simulink model "sysgenQAM16"  (Simulink 7.3)
settings: Solver=ode45  StartTime=0.0  StopTime=5000  RelTol=1e-3
PreLoadFcn:
  | xlrequire('PreLoadFcn')
values from neighbouring files (symbols this model uses):
  hh = hh1/max(hh1)    [sysgenCostasLoop_PreLoadFcn.m]
  j = find(xLabel==')')    [sdspfscope2_r13.m]
  k = (k-1)*3+2    [sdspfscope2_r13.m]
  mu = xfix({xlSigned, 18, 15, xlRound, xlSaturate}, mu)    [lmsErr.m]
undefined symbols (not defined in the file or in its folder): chan, k_i0, k_p0, xlipgetpartsetting, xlsfunxy
libraries: xbsIndex_r4 x263, dspmlti4 x2, dspsigops x2, dspbuff3 x1, xbsCopyrightNotice_r4 x1, dspobslib x1, simulink x1, dspsnks4 x1
(part 1 of 4)
settings Model: Creator=alexc  LastModifiedBy=douangp  ExtModeTrigMode=oneshot  ExtModeArmWhenConnect=off
settings DataIOCC: LimitDataPoints=off  SignalLoggingName=sigsOut
settings OptimizationCC: BlockReduction=off  BooleanDataType=off  InlineInvariantSignals=on  InitFltsAndDblsToZero=on
settings DebuggingCC: SaveWithParameterizedLinksMsg=none  SignalResolutionControl=TryResolveAllWithWarning  SolverPrmCheckMsg=none  MultiTaskDSMMsg=warning  MultiTaskCondExecSysMsg=none  StrictBusMsg=None
settings HardwareCC: TargetUnknown=on
settings RTWCC: IncludeERTFirstTime=on
settings GRTTargetCC: TargetFcnLib=ansi_tfl_tmw.mat

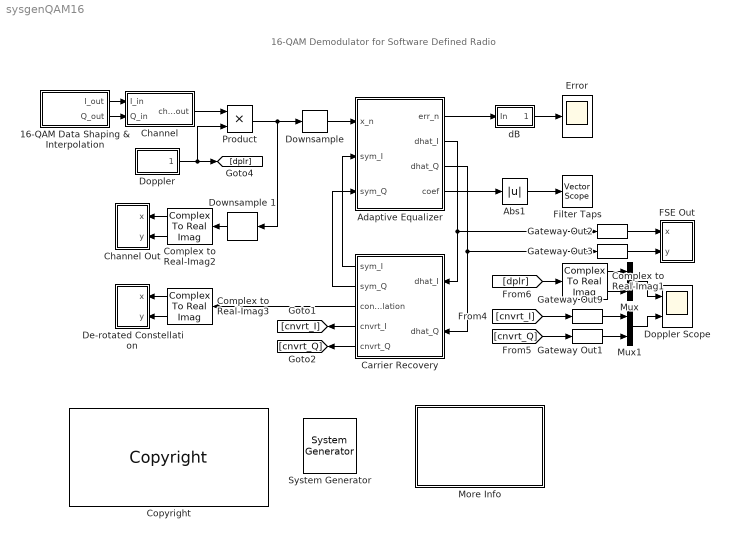
== system sysgenQAM16 ==
  note: 16-QAM Demodulator for Software Defined Radio
  " System Generator" : xbsIndex_r4/ System Generator  Tag=genX  SystemSampleTime=-1  xilinxfamily=virtex6  part=xc6vlx240t  speed=-1  package=ff784  synthesis_tool=XST  clock_wrapper=Clock Enables  directory=./netlist  testbench=off  simulink_period=1  sysclk_period=50  dcm_input_clock_period=100  incr_netlist=off  trim_vbits=Everywhere in SubSystem  dbl_ovrd=According to Block Masks  core_generation=According to Block Masks  run_coregen=off  deprecated_control=off  eval_field=0  block_type=sysgen
      settings: block_version=9.1-beta
  16-QAM Data Shaping & Interpolation : Subsystem
  Abs1 : Abs  SaturateOnIntegerOverflow=on
  Adaptive Equalizer : Subsystem
  Carrier Recovery : Subsystem
  Channel : Subsystem
  Channel Out : Subsystem  LoadFcn=xlsfunxy([],[],[],'LoadBlock')  StartFcn=xlsfunxy([],[],[],'Start')  StopFcn=xlsfunxy([],[],[],'Stop')  mask(My XY scope.){xmin=-2.25, xmax=2.25, ymin=-2.25, ymax=2.25, refresh=800, style='.', st=-1}
      mask prompts: xmin "x-min:"; xmax "x-max:"; ymin "y-min:"; ymax "y-max:"; refresh "Refresh rate"; style "Line/Marker style"; st "Sample time:"
      mask help: XY scope using MATLAB graph window. First input is used as time base. Enter plotting ranges.
      settings: CopyFcn=xlsfunxy([],[],[],'CopyBlock')  DeleteFcn=xlsfunxy([],[],[],'DeleteBlock')  NameChangeFcn=xlsfunxy([],[],[],'NameChange')
      mask Help: This block can be used to explore limit cycles. Look at the m-file xlsfunxy.m to see how it works.
      mask Display: plot([.05 .95 .95 .05 .05],[.45 .45 .95 .95 .45], 0.5+cos(0:0.1:2*pi)*0.3,0.7+sin(0:0.1:2*pi)*0.2)
  Complex to Real-Imag1 : ComplexToRealImag
  Complex to Real-Imag2 : ComplexToRealImag
  Complex to Real-Imag3 : ComplexToRealImag
  Copyright : xbsCopyrightNotice_r4/Copyright  copyrighttext="Copyright (c) 2009  by  Xilinx, Inc. All rights reserved.<br><br>This file contains proprietary, confidential information of Xilinx, Inc., is distributed under licensefrom Xilinx, Inc., and may be used, copied and/or disclosed only pursuant to the terms of a valid licenseagreement with Xilinx, Inc. Xilinx hereby grants you a license to use this file solely for design,simulation, implementation and creation of design files limited to Xilinx devices or technologies. Use with non-Xilinx devices or technologies is expressly prohibited and immediately terminates your license unless covered by a separate agreement.<br><br>Xilinx is providing this design, code, or information \"as-is\" solely for use in developing programs and solutions for Xilinx devices, with no obligation on the part of Xilinx to provide support. By providingthis design, code, or information as one possible implementation of this feature, application or standard,Xilinx is making no representation that this implementation is free from any claims of infringement. Youare responsible for obtaining any rights you may require for your implementation. Xilinx expressly disclaimsany warranty whatsoever with respect to the adequacy of the implementation, including but not limited to anywarranties or representations that this implementation is free from claims of infringement, implied warrantiesof merchantability or fitness for a particular purpose.<br><br>Xilinx products are not intended for use in life support appliances, devices, or systems. Use in such applications is expressly prohibited.<br><br>Any modifications that are made to the Source Code are done at the user's sole risk and will be unsupported.<br><br>This copyright and support notice must be retained as part of this text at all times. (c) Copyright 1995-2009 Xilinx, Inc. All rights reserved."  block_type=copyright
      settings: block_version=10.1.00
      settings: infoedit=|
      | Copyright(C) 2008 by  Xilinx, Inc. All rights reserved.<br>
      | <br>
      | This file contains proprietary, confidential information of Xilinx, Inc., is distributed under license
      | from Xilinx, Inc., and may be used, copied and/or disclosed only pursuant to the terms of a valid license
      | agreement with Xilinx, Inc. Xilinx hereby grants you a license to use this file solely for design,
      | simulation, implementation and creation of design files limited to Xilinx devices or technologies. Use
      | with non-Xilinx devices or technologies is expressly prohibited and immediately terminates your license
      | unless covered by a separate agreement.<br>
      | <br>
      | Xilinx is providing this design, code, or information "as-is" solely for use in developing programs and
      | solutions for Xilinx devices, with no obligation on the part of Xilinx to provide support. By providing
      | this design, code, or information as one possible implementation of this feature, application or standard,
      | Xilinx is making no representation that this implementation is free from any claims of infringement. You
      | are responsible for obtaining any rights you may require for your implementation. Xilinx expressly disclaims
      | any warranty whatsoever with respect to the adequacy of the implementation, including but not limited to any
      | warranties or representations that this implementation is free from claims of infringement, implied warranties
      | of merchantability or fitness for a particular purpose.<br>
      | <br>
      | Xilinx products are not intended for use in life support appliances, devices, or systems. Use in such
      | applications is expressly prohibited.<br>
      | <br>
      | Any modifications that are made to the Source Code are done at the user's sole risk and will be unsupported.<br>
      | <br>
      | This copyright and support notice must be retained as part of this text at all times.
      | (c) Copyright 1995-2008 Xilinx, Inc. All rights reserved.
  De-rotated Constellation : Subsystem  LoadFcn=xlsfunxy([],[],[],'LoadBlock')  StartFcn=xlsfunxy([],[],[],'Start')  StopFcn=xlsfunxy([],[],[],'Stop')  mask(My XY scope.){xmin=-1.5, xmax=1.5, ymin=-1.5, ymax=1.5, refresh=800, style='.', st=-1}
      mask prompts: xmin "x-min:"; xmax "x-max:"; ymin "y-min:"; ymax "y-max:"; refresh "Refresh rate"; style "Line/Marker style"; st "Sample time:"
      mask help: XY scope using MATLAB graph window. First input is used as time base. Enter plotting ranges.
      settings: CopyFcn=xlsfunxy([],[],[],'CopyBlock')  DeleteFcn=xlsfunxy([],[],[],'DeleteBlock')  NameChangeFcn=xlsfunxy([],[],[],'NameChange')
      mask Help: This block can be used to explore limit cycles. Look at the m-file xlsfunxy.m to see how it works.
      mask Display: plot([.05 .95 .95 .05 .05],[.45 .45 .95 .95 .45], 0.5+cos(0:0.1:2*pi)*0.3,0.7+sin(0:0.1:2*pi)*0.2)
  Doppler : Subsystem
  Doppler Scope : Scope  NumInputPorts=2
      settings: TimeRange=4000  YMin=-1~-1  YMax=1~1
  "Downsample " : dspsigops/Downsample  N=2  phase=0  ic=0  smode=Allow multirate  fmode=Maintain input frame size
  Downsample 1 : dspsigops/Downsample  N=4  phase=0  ic=0  smode=Allow multirate  fmode=Maintain input frame size
  Error : Scope
      settings: TimeRange=500  YMin=-60  YMax=-22.5
  FSE Out : Subsystem  LoadFcn=xlsfunxy([],[],[],'LoadBlock')  StartFcn=xlsfunxy([],[],[],'Start')  StopFcn=xlsfunxy([],[],[],'Stop')  mask(My XY scope.){xmin=-2.25, xmax=2.25, ymin=-2.25, ymax=2.25, refresh=800, style='.', st=-1}
      mask prompts: xmin "x-min:"; xmax "x-max:"; ymin "y-min:"; ymax "y-max:"; refresh "Refresh rate"; style "Line/Marker style"; st "Sample time:"
      mask help: XY scope using MATLAB graph window. First input is used as time base. Enter plotting ranges.
      settings: CopyFcn=xlsfunxy([],[],[],'CopyBlock')  DeleteFcn=xlsfunxy([],[],[],'DeleteBlock')  NameChangeFcn=xlsfunxy([],[],[],'NameChange')
      mask Help: This block can be used to explore limit cycles. Look at the m-file xlsfunxy.m to see how it works.
      mask Display: plot([.05 .95 .95 .05 .05],[.45 .45 .95 .95 .45], 0.5+cos(0:0.1:2*pi)*0.3,0.7+sin(0:0.1:2*pi)*0.2)
  Filter Taps : dspsnks4/Vector Scope  DialogController=dspdialog.VectorScope  DialogControllerArgs=DataTag3  ScopeProperties=on  Domain=User-defined  HorizSpan=1  DisplayProperties=off  AxisGrid=on  Memory=off  FrameNumber=on  AxisLegend=off  AxisZoom=on  OpenScopeAtSimStart=on  OpenScopeImmediately=off  FigPos=[66 260 329 270]  AxisProperties=off  XUnits=Hertz  XRange=[0...Fs/2]  InheritXIncr=on  XIncr=1  XLabel=Samples  XLimit=Auto  XMin=0  XMax=1  XStart=0  YUnits=dB  YLabel=Filter Coefficients  LineProperties=off  LineDisables=on  LineStyles=:  LineMarkers=.  LineColors=[0 0 1]  XAxisParamsVer=6.8
      settings: YMin=0.00597900340780036  YMax=1.03689353636578
  Gateway Out{1..3,9} (4 alike) : xbsIndex_r4/Gateway Out  hdl_port=off  timing_constraint=None  locs_specified=off  LOCs={}  block_type=gatewayout
      settings: infoedit="Gateway out block.  Converts Xilinx fixed point inputs into ouputs of type Simulink integer, double, or fixed point.<P><P>Hardware notes:  In hardware these blocks become top level output ports or are discarded, depending on how they are configured."  xl_area=[0 0 0 0 0 0 0]  block_version=VER_STRING_GOES_HERE
  More Info : Subsystem
      mask Display: disp('Double click\n for\n more information.')
  Mux : Mux  Inputs=2
  Mux1 : Mux  Inputs=2
  Product : Product  OutDataType=sfix(16)  OutScaling=2^0  SaturateOnIntegerOverflow=on  InputSameDT=on  OutDataTypeStr=Inherit: Same as first input
  dB : Subsystem
  wires:
  16-QAM Data Shaping & Interpolation/1(I_out) -> Channel/1(I_in)
  "Downsample "/1 -> Adaptive Equalizer/1(x_n)
  16-QAM Data Shaping & Interpolation/2(Q_out) -> Channel/2(Q_in)
  Channel/1(chan_out) -> Product/1
  dB/1(Out) -> Error/1
  Gateway Out9/1 -> Mux1/1
  Gateway Out1/1 -> Mux1/2
  Mux1/1 -> Doppler Scope/2
  Complex to Real-Imag1/2 -> Mux/2
  Complex to Real-Imag1/1 -> Mux/1
  Mux/1 -> Doppler Scope/1
  [cnvrt_Q] -> Gateway Out1/1
  [dplr] -> Complex to Real-Imag1/1
  Doppler/1(doppler) -> [dplr], Product/2
  [cnvrt_I] -> Gateway Out9/1
  Adaptive Equalizer/2(dhat_I) -> Carrier Recovery/1(dhat_I), Gateway Out2/1
  Adaptive Equalizer/3(dhat_Q) -> Carrier Recovery/2(dhat_Q), Gateway Out3/1
  Carrier Recovery/1(sym_I) -> Adaptive Equalizer/2(sym_I)
  Carrier Recovery/2(sym_Q) -> Adaptive Equalizer/3(sym_Q)
  Carrier Recovery/4(cnvrt_I) -> [cnvrt_I]
  Carrier Recovery/5(cnvrt_Q) -> [cnvrt_Q]
  Complex to Real-Imag3/1 -> De-rotated Constellation/1(x)
  Complex to Real-Imag3/2 -> De-rotated Constellation/2(y)
  Carrier Recovery/3(constellation) -> Complex to Real-Imag3/1
  Product/1 -> "Downsample "/1, Downsample 1/1
  Adaptive Equalizer/1(err_n) -> dB/1(In)
  Adaptive Equalizer/4(coef) -> Abs1/1
  Abs1/1 -> Filter Taps/1
  Downsample 1/1 -> Complex to Real-Imag2/1
  Complex to Real-Imag2/2 -> Channel Out/2(y)
  Complex to Real-Imag2/1 -> Channel Out/1(x)
  Gateway Out2/1 -> FSE Out/1(x)
  Gateway Out3/1 -> FSE Out/2(y)

== system sysgenQAM16/16-QAM Data Shaping & Interpolation ==
  Complex to Real-Imag5 : ComplexToRealImag
  "FIR  Interpolation " : dspmlti4/FIR Interpolation  DialogController=dspdialog.FIRInterpolation  DialogControllerArgs=DataTag1  h=[hh]  L=4  framing=Maintain input frame size  outputBufInitCond=0  roundingMode=Floor  overflowMode=off  FilterSource=Specify via dialog  FilterObject=Hm_firinterp
  FIR  Interpolation 1 : dspmlti4/FIR Interpolation  DialogController=dspdialog.FIRInterpolation  DialogControllerArgs=DataTag2  h=[hh]  L=4  framing=Maintain input frame size  outputBufInitCond=0  roundingMode=Floor  overflowMode=off  FilterSource=Specify via dialog  FilterObject=Hm_firinterp
  QAM16 Source : Subsystem
  I_out : Outport  OutDataType=sfix(16)  OutScaling=2^0
  Q_out : Outport  Port=2  OutDataType=sfix(16)  OutScaling=2^0
  wires:
  Complex to Real-Imag5/1 -> "FIR  Interpolation "/1
  Complex to Real-Imag5/2 -> FIR  Interpolation 1/1
  QAM16 Source/1(random_data) -> Complex to Real-Imag5/1
  "FIR  Interpolation "/1 -> I_out/1
  FIR  Interpolation 1/1 -> Q_out/1

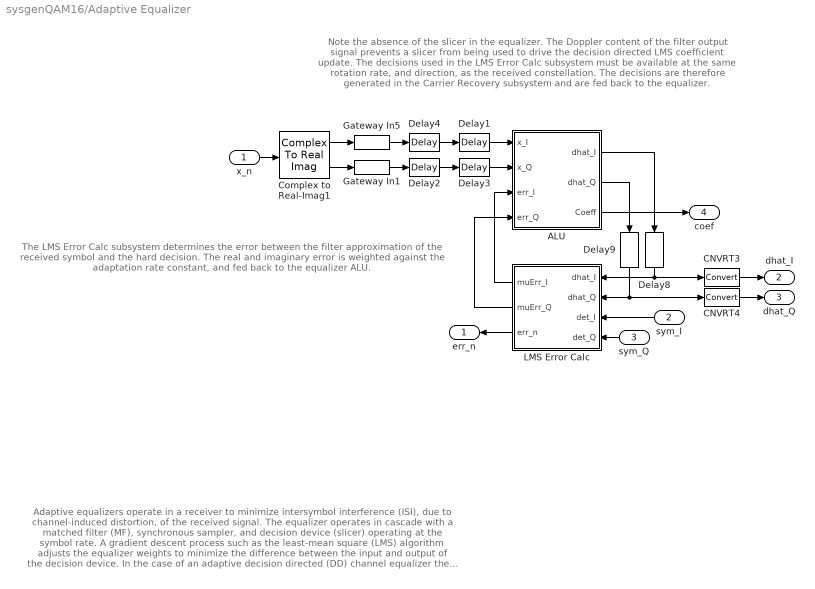
== system sysgenQAM16/Adaptive Equalizer ==
  note: Adaptive equalizers operate in a receiver to minimize intersymbol interference (ISI), due to
      | channel-induced distortion, of the received signal. The equalizer operates in cascade with
      | a matched filter (MF), synchronous sampler, and decision device (slicer) operating at the
      | symbol rate. A gradient descent process such as the least-mean square (LMS) algorithm
      | adjusts the equalizer weights to minimize the difference between the input and output of
      | the decision device.
      |
      | In the case of an adaptive decision directed (DD) channel equalizer the desired signal is
      | produced by utilizing the known structure of the system alphabet.  A 8-tap decision directed
      | equalizer using an LMS coefficient update is used in this model. The input samples are
      | complex valued quantities as are the filter weights and the output signal.
      |
      | A fractionally spaced equalizer (FSE) sampling at a rate of two samples per symbol is
      | used to avoid aliasing.  The equalizer is a multirate structure that is most efficiently
      | implemented using a polyphase decimator architecture.  For this model, two
      | polyphase arms are used.
      |
      | Additional information on adaptive equalizers and FSE can be found at:
      |
      | Haykin, S. "Adaptive Filter Theory"  Prentice Hall, New Jersey, 1996.
      |
      | J.R. Treichler, I. Fijalkow, and C.R. Johnson, Jr.  "Fractionally Spaced
      | Equalizers"  IEEE Signal Processing Magazine, May 1996, pp. 65-81.
  note: The LMS Error Calc subsystem determines
      | the error between the filter approximation of
      | the received symbol and the hard decision.
      | The real and imaginary error is weighted
      | against the adaptation rate constant, and fed
      | back to the equalizer ALU.
  note: Note the absence of the slicer in the equalizer.  The Doppler content
      | of the filter output signal prevents a slicer from being used to drive the
      | decision directed LMS coefficient update.  The decisions used in the
      | LMS Error Calc subsystem must be available at the same rotation rate,
      | and direction, as the received constellation.   The decisions are
      | therefore generated in the Carrier Recovery subsystem and are fed
      | back to the equalizer.
  x_n : Inport  OutDataType=sfix(16)  OutScaling=2^0
  sym_I : Inport  Port=2  OutDataType=sfix(16)  OutScaling=2^0
  sym_Q : Inport  Port=3  OutDataType=sfix(16)  OutScaling=2^0
  ALU : Subsystem
  CNVRT3 : xbsIndex_r4/Convert  arith_type="Signed  (2's comp)"  n_bits=18  bin_pt=14  quantization="Round  (unbiased: +/- Inf)"  overflow=Wrap  latency=0  dbl_ovrd=off  pipeline=off  block_type=convert
      settings: infoedit=The input is presented at the output after quantization and overflow effects.<P><P>Hardware notes: Additional hardware is used when rounding or saturation is selected and output width is less than the input width.  xl_area=[10 0 0 20 0 0 0]  block_version=VER_STRING_GOES_HERE
  CNVRT4 : xbsIndex_r4/Convert  arith_type="Signed  (2's comp)"  n_bits=18  bin_pt=14  quantization="Round  (unbiased: +/- Inf)"  overflow=Wrap  latency=0  dbl_ovrd=off  pipeline=off  block_type=convert
      settings: infoedit=The input is presented at the output after quantization and overflow effects.<P><P>Hardware notes: Additional hardware is used when rounding or saturation is selected and output width is less than the input width.  xl_area=[10 0 0 20 0 0 0]  block_version=VER_STRING_GOES_HERE
  Complex to Real-Imag1 : ComplexToRealImag
  Delay{1..4} (4 alike) : xbsIndex_r4/Delay  en=off  latency=1  dbl_ovrd=off  reg_retiming=off  block_type=delay
      settings: infoedit="Delay line having  configurable length.<P><P>Hardware notes: A delay line is a chain, each link of which is an SRL16 followed by a flip-flop. If register retiming is enabled, the delay line is a chain of flip-flops."  xl_area=[8 16 0 0 0 0 0]  block_version=VER_STRING_GOES_HERE
  Delay8 : xbsIndex_r4/Delay  en=off  latency=k-7  dbl_ovrd=off  reg_retiming=off  block_type=delay
      settings: infoedit="Delay line having  configurable length.<P><P>Hardware notes: A delay line is a chain, each link of which is an SRL16 followed by a flip-flop. If register retiming is enabled, the delay line is a chain of flip-flops."  xl_area=[12 24 0 24 0 0 0]  block_version=VER_STRING_GOES_HERE
  Delay9 : xbsIndex_r4/Delay  en=off  latency=k-7  dbl_ovrd=off  reg_retiming=off  block_type=delay
      settings: infoedit="Delay line having  configurable length.<P><P>Hardware notes: A delay line is a chain, each link of which is an SRL16 followed by a flip-flop. If register retiming is enabled, the delay line is a chain of flip-flops."  xl_area=[12 24 0 24 0 0 0]  block_version=VER_STRING_GOES_HERE
  Gateway In1 : xbsIndex_r4/Gateway In  arith_type="Signed  (2's comp)"  n_bits=xn_ni  bin_pt=xn_nf  quantization="Round  (unbiased: +/- Inf)"  overflow=Saturate  period=2  dbl_ovrd=off  timing_constraint=None  locs_specified=off  LOCs={}  block_type=gatewayin
      settings: infoedit="Gateway in block.  Converts inputs of type Simulink integer, double and fixed point to  Xilinx fixed point type.<P><P>Hardware notes:  In hardware these blocks become top level input ports."  xl_area=[0 0 0 0 16 0 0]  block_version=VER_STRING_GOES_HERE
  Gateway In5 : xbsIndex_r4/Gateway In  arith_type="Signed  (2's comp)"  n_bits=xn_ni  bin_pt=xn_nf  quantization="Round  (unbiased: +/- Inf)"  overflow=Saturate  period=2  dbl_ovrd=off  timing_constraint=None  locs_specified=off  LOCs={}  block_type=gatewayin
      settings: infoedit="Gateway in block.  Converts inputs of type Simulink integer, double and fixed point to  Xilinx fixed point type.<P><P>Hardware notes:  In hardware these blocks become top level input ports."  xl_area=[0 0 0 0 16 0 0]  block_version=VER_STRING_GOES_HERE
  LMS Error Calc : Subsystem
  err_n : Outport  OutDataType=sfix(16)  OutScaling=2^0
  dhat_I : Outport  Port=2  OutDataType=sfix(16)  OutScaling=2^0
  dhat_Q : Outport  Port=3  OutDataType=sfix(16)  OutScaling=2^0
  coef : Outport  Port=4  OutDataType=sfix(16)  OutScaling=2^0
  wires:
  ALU/2(dhat_Q) -> Delay9/1
  Complex to Real-Imag1/1 -> Gateway In5/1
  Complex to Real-Imag1/2 -> Gateway In1/1
  Gateway In5/1 -> Delay4/1
  Gateway In1/1 -> Delay2/1
  x_n/1 -> Complex to Real-Imag1/1
  Delay4/1 -> Delay1/1
  Delay2/1 -> Delay3/1
  Delay1/1 -> ALU/1(x_I)
  Delay3/1 -> ALU/2(x_Q)
  LMS Error Calc/3(err_n) -> err_n/1
  Delay9/1 -> LMS Error Calc/2(dhat_Q), CNVRT4/1
  sym_I/1 -> LMS Error Calc/3(det_I)
  sym_Q/1 -> LMS Error Calc/4(det_Q)
  LMS Error Calc/1(muErr_I) -> ALU/3(err_I)
  LMS Error Calc/2(muErr_Q) -> ALU/4(err_Q)
  ALU/1(dhat_I) -> Delay8/1
  Delay8/1 -> LMS Error Calc/1(dhat_I), CNVRT3/1
  CNVRT3/1 -> dhat_I/1
  CNVRT4/1 -> dhat_Q/1
  ALU/3(Coeff) -> coef/1

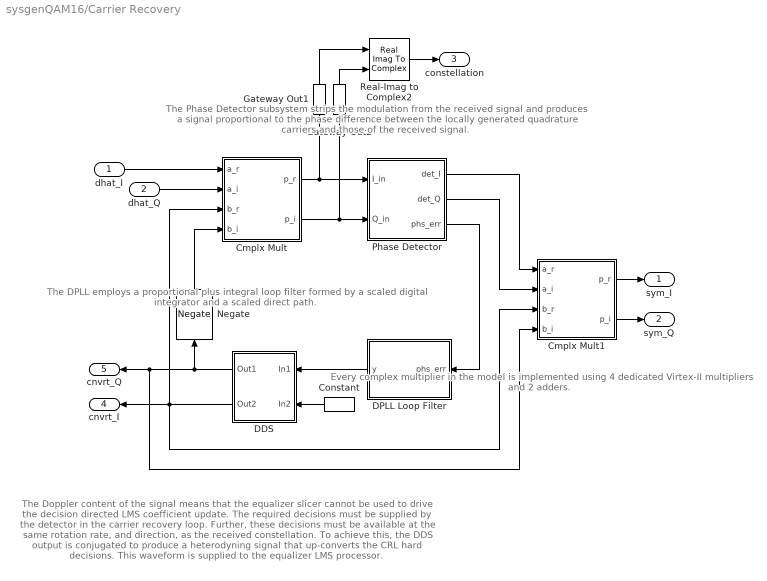
== system sysgenQAM16/Carrier Recovery ==
  note: Every complex multiplier in the model is
      | implemented using 4 dedicated Virtex-II
      | multipliers and 2 adders.
  note: The Doppler content of the signal means that the equalizer slicer cannot be used
      | to drive the decision directed LMS coefficient update.  The required decisions must
      | be supplied by the detector in the carrier recovery loop.  Further, these decisions
      | must be available at the same rotation rate, and direction, as the received constellation.
      | To achieve this, the DDS output is conjugated to produce a heterodyning signal
      | that up-converts the CRL hard decisions. This waveform is supplied to the equalizer
      | LMS processor.
  note: The Phase Detector subsystem strips the modulation
      | from the received signal and produces a signal proportional
      | to the phase difference between the locally generated
      | quadrature carriers and those of the received signal.
  note: The DPLL employs a proportional plus integral
      | loop filter formed by a scaled digital integrator
      | and a scaled direct path.
  dhat_I : Inport  OutDataType=sfix(16)  OutScaling=2^0
  dhat_Q : Inport  Port=2  OutDataType=sfix(16)  OutScaling=2^0
  Cmplx Mult : Subsystem
  Cmplx Mult1 : Subsystem
  Constant : xbsIndex_r4/Constant  arith_type=Boolean  const=1  n_bits=1  bin_pt=0  explicit_period=off  period=1  equ=P=C  opselect=C  inp2=PCIN>>17  opr=+  inp1=P  carry=CIN  dbl_ovrd=off  block_type=constant
      settings: block_version=VER_STRING_GOES_HERE
  DDS : Subsystem
  DPLL Loop Filter : Subsystem
  Gateway Out1 : xbsIndex_r4/Gateway Out  hdl_port=on  timing_constraint="Data Rate;  Set 'FAST' Attribute"  locs_specified=off  LOCs={}  block_type=gatewayout
      settings: infoedit="Gateway out block.  Converts Xilinx fixed point inputs into ouputs of type Simulink integer, double, or fixed point.<P><P>Hardware notes:  In hardware these blocks become top level output ports or are discarded, depending on how they are configured."  xl_area=[0 0 0 0 36 0 0]  block_version=VER_STRING_GOES_HERE
  Gateway Out2 : xbsIndex_r4/Gateway Out  hdl_port=on  timing_constraint="Data Rate;  Set 'FAST' Attribute"  locs_specified=off  LOCs={}  block_type=gatewayout
      settings: infoedit="Gateway out block.  Converts Xilinx fixed point inputs into ouputs of type Simulink integer, double, or fixed point.<P><P>Hardware notes:  In hardware these blocks become top level output ports or are discarded, depending on how they are configured."  xl_area=[0 0 0 0 36 0 0]  block_version=VER_STRING_GOES_HERE
  Negate : xbsIndex_r4/Negate  precision=Full  arith_type=Unsigned  n_bits=8  bin_pt=2  quantization=Truncate  overflow=Wrap  en=off  latency=0  dbl_ovrd=off  block_type=negate
      settings: xl_area=[9 0 0 17 0 0 0]  block_version=VER_STRING_GOES_HERE
  Phase Detector : Subsystem
  Real-Imag to Complex2 : RealImagToComplex
  sym_I : Outport  OutDataType=sfix(16)  OutScaling=2^0
  sym_Q : Outport  Port=2  OutDataType=sfix(16)  OutScaling=2^0
  constellation : Outport  Port=3  OutDataType=sfix(16)  OutScaling=2^0
  cnvrt_I : Outport  Port=4  OutDataType=sfix(16)  OutScaling=2^0
  cnvrt_Q : Outport  Port=5  OutDataType=sfix(16)  OutScaling=2^0
  wires:
  Cmplx Mult/1(p_r) -> Gateway Out1/1, Phase Detector/1(I_in)
  dhat_Q/1 -> Cmplx Mult/2(a_i)
  dhat_I/1 -> Cmplx Mult/1(a_r)
  Cmplx Mult/2(p_i) -> Gateway Out2/1, Phase Detector/2(Q_in)
  Gateway Out1/1 -> Real-Imag to Complex2/1
  Gateway Out2/1 -> Real-Imag to Complex2/2
  Real-Imag to Complex2/1 -> constellation/1
  Cmplx Mult1/2(p_i) -> sym_Q/1
  Phase Detector/3(phs_err) -> DPLL Loop Filter/1(phs_err)
  Phase Detector/1(det_I) -> Cmplx Mult1/1(a_r)
  Phase Detector/2(det_Q) -> Cmplx Mult1/2(a_i)
  Cmplx Mult1/1(p_r) -> sym_I/1
  DDS/2(Out2) -> Cmplx Mult/3(b_r), cnvrt_I/1, Cmplx Mult1/3(b_r)
  DDS/1(Out1) -> cnvrt_Q/1, Cmplx Mult1/4(b_i), Negate/1
  DPLL Loop Filter/1(y) -> DDS/1(In1)
  Constant/1 -> DDS/2(In2)
  Negate/1 -> Cmplx Mult/4(b_i)

== system sysgenQAM16/Channel ==
  I_in : Inport  OutDataType=sfix(16)  OutScaling=2^0
  Q_in : Inport  Port=2  OutDataType=sfix(16)  OutScaling=2^0
  Channel : Subsystem
  Channel1 : Subsystem
  Gain : Gain  Gain=j  ParameterDataType=sfix(16)  ParameterScaling=2^0  OutDataType=sfix(16)  OutScaling=2^0  SaturateOnIntegerOverflow=on  OutDataTypeStr=Inherit: Same as input  ParamDataTypeStr=Inherit: Same as input
  Sum : Sum  OutDataType=sfix(16)  OutScaling=2^0  SaturateOnIntegerOverflow=on  InputSameDT=on  OutDataTypeStr=Inherit: Same as first input
  chan_out : Outport  OutDataType=sfix(16)  OutScaling=2^0
  wires:
  Gain/1 -> Sum/2
  Channel/1(y_n) -> Sum/1
  Channel1/1(y_n) -> Gain/1
  I_in/1 -> Channel/1(x_n)
  Q_in/1 -> Channel1/1(x_n)
  Sum/1 -> chan_out/1

== system sysgenQAM16/Channel Out ==
  x : Inport  OutDataType=sfix(16)  OutScaling=2^0
  y : Inport  Port=2  OutDataType=sfix(16)  OutScaling=2^0
  Mux : Mux  Inputs=2
  xlsfunxy : S-Function  FunctionName=xlsfunxy  Parameters=[xmin xmax ymin ymax],refresh,style,st  EnableBusSupport=off
  wires:
  Mux/1 -> xlsfunxy/1
  x/1 -> Mux/1
  y/1 -> Mux/2

== system sysgenQAM16/De-rotated Constellation ==
  x : Inport  OutDataType=sfix(16)  OutScaling=2^0
  y : Inport  Port=2  OutDataType=sfix(16)  OutScaling=2^0
  Mux : Mux  Inputs=2
  xlsfunxy : S-Function  FunctionName=xlsfunxy  Parameters=[xmin xmax ymin ymax],refresh,style,st  EnableBusSupport=off
  wires:
  Mux/1 -> xlsfunxy/1
  x/1 -> Mux/1
  y/1 -> Mux/2

== system sysgenQAM16/Doppler ==
  DSP Constant : dspobslib/DSP Constant  SystemSampleTime=-1  Value=1  SampleMode=Discrete  discreteOutput=Sample-based  continuousOutput=Sample-based  sampTime=1  framePeriod=1  dataType=Inherit from 'Constant value'  isSigned=on  wordLen=16  udDataType=sfix(16)  fracBitsMode=Best precision  numFracBits=15  InterpretAs1D=off  Ts=1  FramebasedOutput=off
  Frequency Delta : simulink/Math Operations/Slider Gain  SystemSampleTime=-1  low=-0.1  gain=0.001  high=0.1
  R:I : RealImagToComplex
  TX Doppler : Subsystem
  Terminator : Terminator
  doppler : Outport  OutDataType=sfix(16)  OutScaling=2^0
  wires:
  TX Doppler/1(Cos) -> R:I/1
  TX Doppler/2(Sin) -> R:I/2
  Frequency Delta/1 -> TX Doppler/1(In1)
  DSP Constant/1 -> Frequency Delta/1
  R:I/1 -> doppler/1
  TX Doppler/3(DDS Theta) -> Terminator/1

== system sysgenQAM16/FSE Out ==
  x : Inport  OutDataType=sfix(16)  OutScaling=2^0
  y : Inport  Port=2  OutDataType=sfix(16)  OutScaling=2^0
  Mux : Mux  Inputs=2
  xlsfunxy : S-Function  FunctionName=xlsfunxy  Parameters=[xmin xmax ymin ymax],refresh,style,st  EnableBusSupport=off
  wires:
  y/1 -> Mux/2
  x/1 -> Mux/1
  Mux/1 -> xlsfunxy/1

== system sysgenQAM16/More Info ==
  note: 16-QAM Demodulator for Software Defined Radio
  note: This design implements an equalized 16-QAM demodulator for use in a software defined
      | radio.  The receiver architecture provides subsystems that demonstrate adaptive channel
      | equalization and carrier tracking on a random QAM data source.
      |
      | In addition to the System Generator demodulator components, the model includes Simulink
      | subsystems that introduce channel effects and Doppler content into the data source.  Scopes
      | are provided at important nodes for analysis purposes.  The operation of receiver is best
      | illustrated with a long simulation duration, so that the points in the de-rotated constellation
      | have sufficient time to converge.
      |
      | Additional information on software radios can be found at:
      |
      | Chris H. Dick, "Design and implementation of high-performance FPGA signal processing
      | datapaths for software-defined radios" VMEbus Systems, August 2001

== system sysgenQAM16/dB ==
  In : Inport  OutDataType=sfix(16)  OutScaling=2^0
  Abs : Abs  SaturateOnIntegerOverflow=on
  Constant : Constant  Value=0  OutDataType=sfix(16)  OutScaling=2^0
  Constant1 : Constant  OutDataType=sfix(16)  OutScaling=2^0
  Constant2 : Constant  OutDataType=sfix(16)  OutScaling=2^0
  Gain1 : Gain  Gain=20  ParameterDataType=sfix(16)  ParameterScaling=2^0  OutDataType=sfix(16)  OutScaling=2^0  SaturateOnIntegerOverflow=on  OutDataTypeStr=Inherit: Same as input  ParamDataTypeStr=Inherit: Same as input
  Multiport Switch : MultiPortSwitch  Inputs=2  SaturateOnIntegerOverflow=on  InputSameDT=on
  Relational Operator : RelationalOperator  Operator===  InputSameDT=on
  Sum : Sum  Inputs=|++  OutDataType=sfix(16)  OutScaling=2^0  SaturateOnIntegerOverflow=on  InputSameDT=on  OutDataTypeStr=Inherit: Same as first input
  log10 : Math  Operator=log10  OutDataType=sfix(16)  OutScaling=2^0  SaturateOnIntegerOverflow=on
  Out : Outport  OutDataType=sfix(16)  OutScaling=2^0
  wires:
  Multiport Switch/1 -> log10/1
  Constant1/1 -> Multiport Switch/3
  Constant/1 -> Relational Operator/1
  Abs/1 -> Multiport Switch/2, Relational Operator/2
  Constant2/1 -> Sum/2
  Sum/1 -> Multiport Switch/1
  Relational Operator/1 -> Sum/1
  Gain1/1 -> Out/1
  In/1 -> Abs/1
  log10/1 -> Gain1/1

== system sysgenQAM16/16-QAM Data Shaping & Interpolation/QAM16 Source ==
  QAM16 - I : Subsystem
  QAM16 -Q : Subsystem
  Real-Imag to Complex : RealImagToComplex
  random_data : Outport  OutDataType=sfix(16)  OutScaling=2^0
  wires:
  Real-Imag to Complex/1 -> random_data/1
  QAM16 -Q/1(Q) -> Real-Imag to Complex/2
  QAM16 - I/1(I) -> Real-Imag to Complex/1

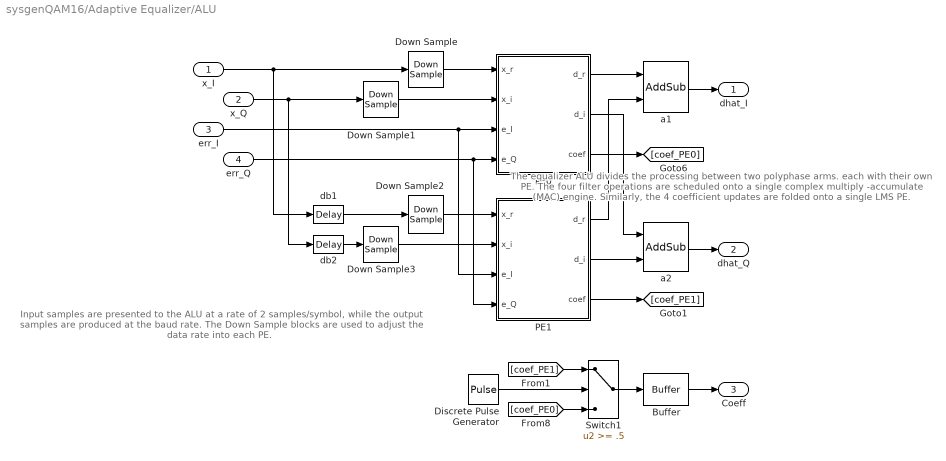
== system sysgenQAM16/Adaptive Equalizer/ALU ==
  note: The equalizer ALU divides the processing between two
      | polyphase arms.  each with their own PE.  The four filter
      | operations are scheduled onto a single complex multiply
      | -accumulate (MAC) engine.  Similarly, the 4 coefficient
      | updates are folded onto a single LMS PE.
  note: Input samples are presented to the ALU at a rate
      | of 2 samples/symbol, while the output samples
      | are produced at the baud rate.  The Down
      | Sample blocks are used to adjust the data rate
      | into each PE.
  x_I : Inport  OutDataType=sfix(16)  OutScaling=2^0
  x_Q : Inport  Port=2  OutDataType=sfix(16)  OutScaling=2^0
  err_I : Inport  Port=3  OutDataType=sfix(16)  OutScaling=2^0
  err_Q : Inport  Port=4  OutDataType=sfix(16)  OutScaling=2^0
  Buffer : dspbuff3/Buffer  N=8  V=0  ic=0
  Discrete Pulse Generator : DiscretePulseGenerator  Amplitude=1  Period=2  PulseWidth=1  PhaseDelay=0  SampleTime=.5
  Down Sample{,1..3} (4 alike) : xbsIndex_r4/Down Sample  sample_ratio=2  sample_phase="Last Value of Frame  (most efficient)"  en=off  latency=2  dbl_ovrd=off  block_type=dsamp
      settings: xl_area=[8 16 0 16 0 0 0]  block_version=VER_STRING_GOES_HERE
  PE0 : Subsystem
  PE1 : Subsystem
  Switch1 : Switch  Threshold=.5  SaturateOnIntegerOverflow=on  InputSameDT=on
  a1 : xbsIndex_r4/AddSub  mode=Addition  use_carryin=off  use_carryout=off  en=off  latency=2  precision=User Defined  arith_type="Signed  (2's comp)"  n_bits=24  bin_pt=20  quantization=Truncate  overflow=Saturate  dbl_ovrd=off  use_behavioral_HDL=on  hw_selection=Fabric  pipelined=off  use_rpm=off  block_type=addsub
      settings: xl_area=[38 50 0 48 0 0 0]  block_version=VER_STRING_GOES_HERE
  a2 : xbsIndex_r4/AddSub  mode=Addition  use_carryin=off  use_carryout=off  en=off  latency=2  precision=User Defined  arith_type="Signed  (2's comp)"  n_bits=24  bin_pt=20  quantization=Truncate  overflow=Saturate  dbl_ovrd=off  use_behavioral_HDL=on  hw_selection=Fabric  pipelined=off  use_rpm=off  block_type=addsub
      settings: xl_area=[38 50 0 48 0 0 0]  block_version=VER_STRING_GOES_HERE
  db1 : xbsIndex_r4/Delay  en=off  latency=1  dbl_ovrd=off  reg_retiming=off  block_type=delay
      settings: infoedit="Delay line having  configurable length.<P><P>Hardware notes: A delay line is a chain, each link of which is an SRL16 followed by a flip-flop. If register retiming is enabled, the delay line is a chain of flip-flops."  xl_area=[8 16 0 0 0 0 0]  block_version=VER_STRING_GOES_HERE
  db2 : xbsIndex_r4/Delay  en=off  latency=1  dbl_ovrd=off  reg_retiming=off  block_type=delay
      settings: infoedit="Delay line having  configurable length.<P><P>Hardware notes: A delay line is a chain, each link of which is an SRL16 followed by a flip-flop. If register retiming is enabled, the delay line is a chain of flip-flops."  xl_area=[8 16 0 0 0 0 0]  block_version=VER_STRING_GOES_HERE
  dhat_I : Outport  OutDataType=sfix(16)  OutScaling=2^0
  dhat_Q : Outport  Port=2  OutDataType=sfix(16)  OutScaling=2^0
  Coeff : Outport  Port=3  OutDataType=sfix(16)  OutScaling=2^0
  wires:
  err_I/1 -> PE0/3(e_I), PE1/3(e_I)
  err_Q/1 -> PE0/4(e_Q), PE1/4(e_Q)
  x_I/1 -> Down Sample/1, db1/1
  x_Q/1 -> Down Sample1/1, db2/1
  Down Sample/1 -> PE0/1(x_r)
  Down Sample1/1 -> PE0/2(x_i)
  PE0/1(d_r) -> a1/1
  PE0/2(d_i) -> a2/1
  a1/1 -> dhat_I/1
  a2/1 -> dhat_Q/1
  db1/1 -> Down Sample2/1
  db2/1 -> Down Sample3/1
  Buffer/1 -> Coeff/1
  PE0/3(coef) -> [coef_PE0]
  Down Sample2/1 -> PE1/1(x_r)
  Down Sample3/1 -> PE1/2(x_i)
  PE1/3(coef) -> [coef_PE1]
  PE1/1(d_r) -> a1/2
  PE1/2(d_i) -> a2/2
  [coef_PE0] -> Switch1/3
  [coef_PE1] -> Switch1/1
  Discrete Pulse Generator/1 -> Switch1/2
  Switch1/1 -> Buffer/1

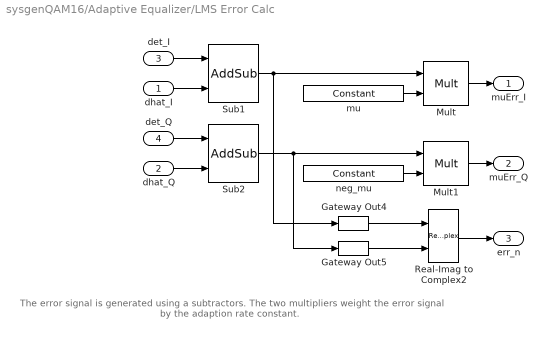
== system sysgenQAM16/Adaptive Equalizer/LMS Error Calc ==
  note: The error signal is generated using a subtractors.  The
      | two multipliers weight  the error signal by the adaption
      | rate constant.
  dhat_I : Inport  OutDataType=sfix(16)  OutScaling=2^0
  dhat_Q : Inport  Port=2  OutDataType=sfix(16)  OutScaling=2^0
  det_I : Inport  Port=3  OutDataType=sfix(16)  OutScaling=2^0
  det_Q : Inport  Port=4  OutDataType=sfix(16)  OutScaling=2^0
  Gateway Out4 : xbsIndex_r4/Gateway Out  hdl_port=off  timing_constraint=None  locs_specified=off  LOCs={}  block_type=gatewayout
      settings: infoedit="Gateway out block.  Converts Xilinx fixed point inputs into ouputs of type Simulink integer, double, or fixed point.<P><P>Hardware notes:  In hardware these blocks become top level output ports or are discarded, depending on how they are configured."  xl_area=[0 0 0 0 0 0 0]  block_version=VER_STRING_GOES_HERE
  Gateway Out5 : xbsIndex_r4/Gateway Out  hdl_port=off  timing_constraint=None  locs_specified=off  LOCs={}  block_type=gatewayout
      settings: infoedit="Gateway out block.  Converts Xilinx fixed point inputs into ouputs of type Simulink integer, double, or fixed point.<P><P>Hardware notes:  In hardware these blocks become top level output ports or are discarded, depending on how they are configured."  xl_area=[0 0 0 0 0 0 0]  block_version=VER_STRING_GOES_HERE
  Mult : xbsIndex_r4/Mult  precision=User Defined  arith_type="Signed  (2's comp)"  n_bits=mu_mult_ni  bin_pt=mu_mult_nf  quantization="Round  (unbiased: +/- Inf)"  overflow=Wrap  en=off  latency=2  dbl_ovrd=off  use_behavioral_HDL=off  opt=Speed  use_embedded=on  optimum_pipeline=off  pipeline=off  use_rpm=off  placement_style=Rectangular shape  block_type=mult
      settings: infoedit=Multiplies two values.<P><P>Hardware notes: To use the internal pipeline stage of the dedicated multiplier you must select 'Pipeline to Greatest Extent Possible'.  xl_area=[105 139 0 97 0 4 0]  block_version=VER_STRING_GOES_HERE
  Mult1 : xbsIndex_r4/Mult  precision=User Defined  arith_type="Signed  (2's comp)"  n_bits=mu_mult_ni  bin_pt=mu_mult_nf  quantization="Round  (unbiased: +/- Inf)"  overflow=Wrap  en=off  latency=2  dbl_ovrd=off  use_behavioral_HDL=off  opt=Speed  use_embedded=on  optimum_pipeline=off  pipeline=off  use_rpm=off  placement_style=Rectangular shape  block_type=mult
      settings: infoedit=Multiplies two values.<P><P>Hardware notes: To use the internal pipeline stage of the dedicated multiplier you must select 'Pipeline to Greatest Extent Possible'.  xl_area=[105 139 0 97 0 4 0]  block_version=VER_STRING_GOES_HERE
  Real-Imag to Complex2 : RealImagToComplex
  Sub1 : xbsIndex_r4/AddSub  mode=Subtraction  use_carryin=off  use_carryout=off  en=off  latency=1  precision=User Defined  arith_type="Signed  (2's comp)"  n_bits=err_ni  bin_pt=err_nf  quantization=Truncate  overflow=Saturate  dbl_ovrd=off  use_behavioral_HDL=on  hw_selection=Fabric  pipelined=off  use_rpm=off  block_type=addsub
      settings: xl_area=[33 29 0 64 0 0 0]  block_version=VER_STRING_GOES_HERE
  Sub2 : xbsIndex_r4/AddSub  mode=Subtraction  use_carryin=off  use_carryout=off  en=off  latency=1  precision=User Defined  arith_type="Signed  (2's comp)"  n_bits=err_ni  bin_pt=err_nf  quantization="Round  (unbiased: +/- Inf)"  overflow=Saturate  dbl_ovrd=off  use_behavioral_HDL=on  hw_selection=Fabric  pipelined=off  use_rpm=off  block_type=addsub
      settings: xl_area=[51 37 0 98 0 0 0]  block_version=VER_STRING_GOES_HERE
  mu : xbsIndex_r4/Constant  arith_type=Signed (2's comp)  const=mu  n_bits=mu_ni  bin_pt=mu_nf  explicit_period=off  period=1  equ=P=C  opselect=C  inp2=PCIN>>17  opr=+  inp1=P  carry=CIN  dbl_ovrd=off  block_type=constant
      settings: block_version=VER_STRING_GOES_HERE
  neg_mu : xbsIndex_r4/Constant  arith_type=Signed (2's comp)  const=-mu  n_bits=mu_ni  bin_pt=mu_nf  explicit_period=off  period=1  equ=P=C  opselect=C  inp2=PCIN>>17  opr=+  inp1=P  carry=CIN  dbl_ovrd=off  block_type=constant
      settings: block_version=VER_STRING_GOES_HERE
  muErr_I : Outport  OutDataType=sfix(16)  OutScaling=2^0
  muErr_Q : Outport  Port=2  OutDataType=sfix(16)  OutScaling=2^0
  err_n : Outport  Port=3  OutDataType=sfix(16)  OutScaling=2^0
  wires:
  Mult/1 -> muErr_I/1
  Mult1/1 -> muErr_Q/1
  neg_mu/1 -> Mult1/2
  mu/1 -> Mult/2
  det_I/1 -> Sub1/1
  dhat_I/1 -> Sub1/2
  det_Q/1 -> Sub2/1
  dhat_Q/1 -> Sub2/2
  Sub1/1 -> Mult/1, Gateway Out4/1
  Sub2/1 -> Mult1/1, Gateway Out5/1
  Real-Imag to Complex2/1 -> err_n/1
  Gateway Out4/1 -> Real-Imag to Complex2/1
  Gateway Out5/1 -> Real-Imag to Complex2/2

== system sysgenQAM16/Carrier Recovery/Cmplx Mult ==
  a_r : Inport  OutDataType=sfix(16)  OutScaling=2^0
  a_i : Inport  Port=2  OutDataType=sfix(16)  OutScaling=2^0
  b_r : Inport  Port=3  OutDataType=sfix(16)  OutScaling=2^0
  b_i : Inport  Port=4  OutDataType=sfix(16)  OutScaling=2^0
  AddSub : xbsIndex_r4/AddSub  mode=Subtraction  use_carryin=off  use_carryout=off  en=off  latency=0  precision=User Defined  arith_type="Signed  (2's comp)"  n_bits=lms_mult_post_add_ni  bin_pt=lms_mult_post_add_nf  quantization=Truncate  overflow=Wrap  dbl_ovrd=off  use_behavioral_HDL=on  hw_selection=Fabric  pipelined=off  use_rpm=on  block_type=addsub
      settings: xl_area=[18 0 0 36 0 0 0]  block_version=VER_STRING_GOES_HERE
  AddSub1 : xbsIndex_r4/AddSub  mode=Addition  use_carryin=off  use_carryout=off  en=off  latency=0  precision=User Defined  arith_type="Signed  (2's comp)"  n_bits=lms_mult_post_add_ni  bin_pt=lms_mult_post_add_nf  quantization=Truncate  overflow=Wrap  dbl_ovrd=off  use_behavioral_HDL=on  hw_selection=Fabric  pipelined=off  use_rpm=on  block_type=addsub
      settings: xl_area=[18 0 0 36 0 0 0]  block_version=VER_STRING_GOES_HERE
  Mult{1..4} (4 alike) : xbsIndex_r4/Mult  precision=User Defined  arith_type="Signed  (2's comp)"  n_bits=lms_mult_ni  bin_pt=lms_mult_nf  quantization=Truncate  overflow=Wrap  en=off  latency=0  dbl_ovrd=off  use_behavioral_HDL=off  opt=Speed  use_embedded=on  optimum_pipeline=off  pipeline=off  use_rpm=on  placement_style=Rectangular shape  block_type=mult
      Mult1 settings: infoedit=Multiplies two values.<P><P>Hardware notes: To use the internal pipeline stage of the dedicated multiplier you must select 'Pipeline to Greatest Extent Possible'.  xl_area=[18 0 0 35 0 1 0]  block_version=VER_STRING_GOES_HERE
      Mult2 settings: infoedit=Multiplies two values.<P><P>Hardware notes: To use the internal pipeline stage of the dedicated multiplier you must select 'Pipeline to Greatest Extent Possible'.  xl_area=[18 0 0 35 0 1 0]  block_version=VER_STRING_GOES_HERE
      Mult3 settings: infoedit=Multiplies two values.<P><P>Hardware notes: To use the internal pipeline stage of the dedicated multiplier you must select 'Pipeline to Greatest Extent Possible'.  xl_area=[17 0 0 34 0 1 0]  block_version=VER_STRING_GOES_HERE
      Mult4 settings: infoedit=Multiplies two values.<P><P>Hardware notes: To use the internal pipeline stage of the dedicated multiplier you must select 'Pipeline to Greatest Extent Possible'.  xl_area=[17 0 0 34 0 1 0]  block_version=VER_STRING_GOES_HERE
  p_r : Outport  OutDataType=sfix(16)  OutScaling=2^0
  p_i : Outport  Port=2  OutDataType=sfix(16)  OutScaling=2^0
  wires:
  AddSub1/1 -> p_i/1
  AddSub/1 -> p_r/1
  Mult3/1 -> AddSub1/2
  Mult2/1 -> AddSub1/1
  Mult1/1 -> AddSub/2
  a_r/1 -> Mult2/1, Mult4/1
  b_i/1 -> Mult2/2, Mult1/2
  b_r/1 -> Mult3/1, Mult4/2
  a_i/1 -> Mult3/2, Mult1/1
  Mult4/1 -> AddSub/1

== system sysgenQAM16/Carrier Recovery/Cmplx Mult1 ==
  a_r : Inport  OutDataType=sfix(16)  OutScaling=2^0
  a_i : Inport  Port=2  OutDataType=sfix(16)  OutScaling=2^0
  b_r : Inport  Port=3  OutDataType=sfix(16)  OutScaling=2^0
  b_i : Inport  Port=4  OutDataType=sfix(16)  OutScaling=2^0
  AddSub : xbsIndex_r4/AddSub  mode=Subtraction  use_carryin=off  use_carryout=off  en=off  latency=0  precision=User Defined  arith_type="Signed  (2's comp)"  n_bits=lms_mult_post_add_ni  bin_pt=lms_mult_post_add_nf  quantization=Truncate  overflow=Wrap  dbl_ovrd=off  use_behavioral_HDL=on  hw_selection=Fabric  pipelined=off  use_rpm=on  block_type=addsub
      settings: xl_area=[18 0 0 36 0 0 0]  block_version=VER_STRING_GOES_HERE
  AddSub1 : xbsIndex_r4/AddSub  mode=Addition  use_carryin=off  use_carryout=off  en=off  latency=0  precision=User Defined  arith_type="Signed  (2's comp)"  n_bits=lms_mult_post_add_ni  bin_pt=lms_mult_post_add_nf  quantization=Truncate  overflow=Wrap  dbl_ovrd=off  use_behavioral_HDL=on  hw_selection=Fabric  pipelined=off  use_rpm=on  block_type=addsub
      settings: xl_area=[18 0 0 36 0 0 0]  block_version=VER_STRING_GOES_HERE
  Mult{1..4} (4 alike) : xbsIndex_r4/Mult  precision=User Defined  arith_type="Signed  (2's comp)"  n_bits=lms_mult_ni  bin_pt=lms_mult_nf  quantization=Truncate  overflow=Wrap  en=off  latency=0  dbl_ovrd=off  use_behavioral_HDL=off  opt=Speed  use_embedded=on  optimum_pipeline=off  pipeline=off  use_rpm=on  placement_style=Rectangular shape  block_type=mult
      settings: infoedit=Multiplies two values.<P><P>Hardware notes: To use the internal pipeline stage of the dedicated multiplier you must select 'Pipeline to Greatest Extent Possible'.  xl_area=[16 0 0 32 0 1 0]  block_version=VER_STRING_GOES_HERE
  p_r : Outport  OutDataType=sfix(16)  OutScaling=2^0
  p_i : Outport  Port=2  OutDataType=sfix(16)  OutScaling=2^0
  wires:
  Mult4/1 -> AddSub/1
  a_i/1 -> Mult1/1, Mult3/2
  b_r/1 -> Mult4/2, Mult3/1
  b_i/1 -> Mult1/2, Mult2/2
  a_r/1 -> Mult4/1, Mult2/1
  Mult1/1 -> AddSub/2
  Mult2/1 -> AddSub1/1
  Mult3/1 -> AddSub1/2
  AddSub/1 -> p_r/1
  AddSub1/1 -> p_i/1

== system sysgenQAM16/Carrier Recovery/DDS ==
  In1 : Inport  OutDataType=sfix(16)  OutScaling=2^0
  In2 : Inport  Port=2  OutDataType=sfix(16)  OutScaling=2^0
  Convert : xbsIndex_r4/Convert  arith_type=Unsigned  n_bits=14  bin_pt=14  quantization=Truncate  overflow=Wrap  latency=0  dbl_ovrd=off  pipeline=off  block_type=convert
      settings: block_version=VER_STRING_GOES_HERE
  "DDS Compiler 4.0 " : xbsIndex_r4/DDS Compiler 4.0   partspresent=Phase_Generator_and_SIN_COS_LUT  dds_clock_rate=100  channels=1  parameter_entry=System_Parameters  spurious_free_dynamic_range=96  frequency_resolution=10000  noise_shaping=Auto  phase_width=28  output_width=6  output_selection=Sine_and_Cosine  negative_sine=off  negative_cosine=off  amplitude_mode=Full_Range  memory_type=Auto  optimization_goal=Auto  dsp48_use=Minimal  latency_configuration=Auto  latency=2  has_phase_out=off  sclr_pin=off  clock_enable=off  rfd=off  rdy=on  channel_pin=off  explicit_period=off  period=1  phase_increment=Programmable  output_frequency1=0  output_frequency2=0  output_frequency3=0  output_frequency4=0  output_frequency5=0  output_frequency6=0  output_frequency7=0  output_frequency8=0  output_frequency9=0  output_frequency10=0  output_frequency11=0  output_frequency12=0  output_frequency13=0  output_frequency14=0  output_frequency15=0  output_frequency16=0  pinc1='0'  pinc2='0'  pinc3='0'  pinc4='0'  pinc5='0'  pinc6='0'  pinc7='0'  pinc8='0'  pinc9='0'  pinc10='0'  pinc11='0'  pinc12='0'  pinc13='0'  pinc14='0'  pinc15='0'  pinc16='0'  phase_offset=None  phase_offset_angles1=0  phase_offset_angles2=0  phase_offset_angles3=0  phase_offset_angles4=0  phase_offset_angles5=0  phase_offset_angles6=0  phase_offset_angles7=0  phase_offset_angles8=0  phase_offset_angles9=0  phase_offset_angles10=0  phase_offset_angles11=0  phase_offset_angles12=0  phase_offset_angles13=0  phase_offset_angles14=0  phase_offset_angles15=0  phase_offset_angles16=0  poff1='0'  poff2='0'  poff3='0'  poff4='0'  poff5='0'  poff6='0'  poff7='0'  poff8='0'  poff9='0'  poff10='0'  poff11='0'  poff12='0'  poff13='0'  poff14='0'  poff15='0'  poff16='0'  por_mode=false  gui_behaviour=Sysgen  ip_name=DDS Compiler  ip_version=4.0  dsptool_ready=true  wrapper_available=true  port_translation_map={ 'ce' => 'en', 'sclr' => 'rst' }  ipcore_xco_need_fpga_part=true  ipcore_fpga_part=xlipgetpartsetting(gcb, {'virtex4', 'xc4vsx35', '-10', 'ff668'})  ipcore_usecache=true  ipcore_useipmodelcache=true  ipcore_verbose=false  block_type=dds_compiler_v4_0
      settings: block_version=11.3
  Register : xbsIndex_r4/Register  init=0  rst=off  en=on  dbl_ovrd=off  block_type=register
  Register1 : xbsIndex_r4/Register  init=0  rst=off  en=on  dbl_ovrd=off  block_type=register
  Reinterpret : xbsIndex_r4/Reinterpret  force_arith_type=on  arith_type="Signed  (2's comp)"  force_bin_pt=off  bin_pt=0  block_type=cast
      settings: infoedit="Changes type of samples without altering their binary representation.<P><P>Hardware notes: In hardware this block costs nothing.<P><P>Example:  Suppose the input is 6 bits wide, signed, with 2 fractional bits, and the output is forced to unsigned with 0 fractional bits.  Then an input of -2.0 (1110.00 in binary 2's complement) becomes an output of 56 (111000 in binary)."  block_version=VER_STRING_GOES_HERE
  Reinterpret1 : xbsIndex_r4/Reinterpret  force_arith_type=off  arith_type="Signed  (2's comp)"  force_bin_pt=on  bin_pt=15  block_type=cast
      settings: infoedit="Changes type of samples without altering their binary representation.<P><P>Hardware notes: In hardware this block costs nothing.<P><P>Example:  Suppose the input is 6 bits wide, signed, with 2 fractional bits, and the output is forced to unsigned with 0 fractional bits.  Then an input of -2.0 (1110.00 in binary 2's complement) becomes an output of 56 (111000 in binary)."  block_version=VER_STRING_GOES_HERE
  Reinterpret2 : xbsIndex_r4/Reinterpret  force_arith_type=off  arith_type="Signed  (2's comp)"  force_bin_pt=on  bin_pt=15  block_type=cast
      settings: infoedit="Changes type of samples without altering their binary representation.<P><P>Hardware notes: In hardware this block costs nothing.<P><P>Example:  Suppose the input is 6 bits wide, signed, with 2 fractional bits, and the output is forced to unsigned with 0 fractional bits.  Then an input of -2.0 (1110.00 in binary 2's complement) becomes an output of 56 (111000 in binary)."  block_version=VER_STRING_GOES_HERE
  Reinterpret3 : xbsIndex_r4/Reinterpret  force_arith_type=on  arith_type=Unsigned  force_bin_pt=off  bin_pt=0  block_type=cast
      settings: infoedit="Changes signal type without altering the binary representation.   You can changed the signal between signed and unsigned, and relocate the binary point.<br><br>Hardware notes: In hardware this block costs nothing.<br><br>Example:  Suppose the input is 6 bits wide, signed, with 2 fractional bits, and the output is forced to unsigned with 0 fractional bits.  Then an input of -2.0 (1110.00 in binary 2's complement) becomes an output of 56 (111000 in binary)."  block_version=VER_STRING_GOES_HERE
  Resource Estimator : xbsIndex_r4/Resource Estimator  Tag=resEstTag  Slices=18  FFs=20  BRAMs=1  LUTs=20  IOBs=0  EBMs=0  TBUFs=0  xl_use_estimator_area=on  est_options=Estimate  xl_estimator_area=[18 20 1 20 0 0 0]  mrp_directory=./sysgenQAM16_DDS_work  simulink_period=1  block_type=resource_estimator
      settings: AttributesFormatString=Resource\nEstimator  block_version=9.1-beta
  Out1 : Outport  OutDataType=sfix(16)  OutScaling=2^0
  Out2 : Outport  Port=2  OutDataType=sfix(16)  OutScaling=2^0
  wires:
  In1/1 -> Convert/1
  Convert/1 -> Reinterpret/1
  Register/1 -> Reinterpret2/1
  Register1/1 -> Reinterpret1/1
  Reinterpret2/1 -> Out1/1
  Reinterpret1/1 -> Out2/1
  "DDS Compiler 4.0 "/2 -> Register/1
  "DDS Compiler 4.0 "/3 -> Register1/1
  Reinterpret/1 -> Reinterpret3/1
  In2/1 -> "DDS Compiler 4.0 "/1
  "DDS Compiler 4.0 "/1 -> Register/2, Register1/2
  Reinterpret3/1 -> "DDS Compiler 4.0 "/2
